simulink library "GAS_MASTER"  (Simulink 8.6)
settings: Solver=ode45  StartTime=0.0  StopTime=10.0  RelTol=1e-3
libraries: cdsEpicsOut x24, cdsFilt x14, cdsFiltCtrl x10, cdsTP x8, VIS_LIB x8, cdsEpicsBinIn x7, cdsEpicsIn x6, cdsFunctionCall x4
(part 1 of 3)
settings Model: Creator=controls  LastModifiedBy=controls

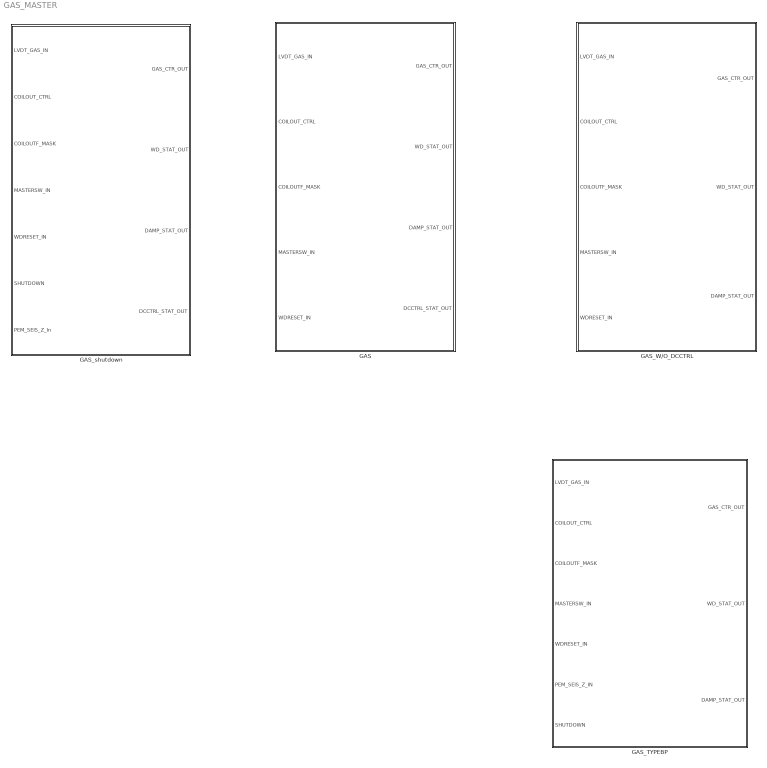
== system GAS_MASTER ==
  GAS : Subsystem
  GAS_TYPEBP : Subsystem
  GAS_W/O_DCCTRL : Subsystem
  GAS_shutdown : Subsystem

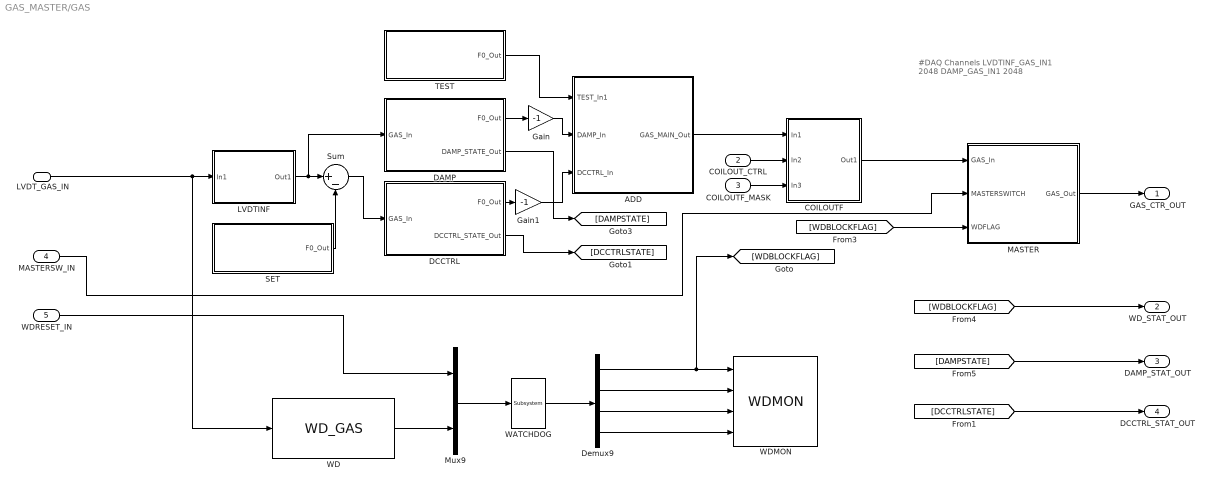
== system GAS_MASTER/GAS ==
  note: #DAQ Channels
      | LVDTINF_GAS_IN1 2048
      | DAMP_GAS_IN1 2048
  LVDT_GAS_IN : Inport
  COILOUT_CTRL : Inport  Port=2
  COILOUTF_MASK : Inport  Port=3
  MASTERSW_IN : Inport  Port=4
  WDRESET_IN : Inport  Port=5
  ADD : Subsystem
  COILOUTF : Subsystem
  DAMP : Subsystem
  DCCTRL : Subsystem
  Demux9 : Demux
  Gain : Gain  Gain=-1
  Gain1 : Gain  Gain=-1
  LVDTINF : Subsystem
  MASTER : Subsystem
  Mux9 : Mux  Inputs=2
  SET : Subsystem
  Sum : Sum  Inputs=|+-
  TEST : Subsystem
  WATCHDOG : cdsFunctionCall/Subsystem  Tag=cdsFunctionCall  Description=inline OSEMWATCHDOG /opt/rtcds/userapps/release/vis/common/src/WATCHDOG.c
      settings: AttributesFormatString=%<Tag>\n%<Description>
  WD : VIS_LIB/WD_GAS
  WDMON : VIS_LIB/WDMON
  GAS_CTR_OUT : Outport
  WD_STAT_OUT : Outport  Port=2
  DAMP_STAT_OUT : Outport  Port=3
  DCCTRL_STAT_OUT : Outport  Port=4
  wires:
  Demux9/2 -> WDMON/2
  Demux9/3 -> WDMON/3
  WD/1 -> Mux9/2
  COILOUTF/1(Out1) -> MASTER/1(GAS_In)
  LVDTINF/1(Out1) -> Sum/1, DAMP/1(GAS_In)
  WATCHDOG/1 -> Demux9/1
  Demux9/4 -> WDMON/4
  Mux9/1 -> WATCHDOG/1
  DAMP/2(DAMP_STATE_Out) -> [DAMPSTATE]
  DAMP/1(F0_Out) -> Gain/1
  MASTERSW_IN/1 -> MASTER/2(MASTERSWITCH)
  [WDBLOCKFLAG] -> WD_STAT_OUT/1
  [DAMPSTATE] -> DAMP_STAT_OUT/1
  [WDBLOCKFLAG] -> MASTER/3(WDFLAG)
  MASTER/1(GAS_Out) -> GAS_CTR_OUT/1
  ADD/1(GAS_MAIN_Out) -> COILOUTF/1(In1)
  Demux9/1 -> [WDBLOCKFLAG], WDMON/1
  LVDT_GAS_IN/1 -> LVDTINF/1(In1), WD/1
  COILOUT_CTRL/1 -> COILOUTF/2(In2)
  COILOUTF_MASK/1 -> COILOUTF/3(In3)
  WDRESET_IN/1 -> Mux9/1
  DCCTRL/1(F0_Out) -> Gain1/1
  DCCTRL/2(DCCTRL_STATE_Out) -> [DCCTRLSTATE]
  [DCCTRLSTATE] -> DCCTRL_STAT_OUT/1
  Sum/1 -> DCCTRL/1(GAS_In)
  TEST/1(F0_Out) -> ADD/1(TEST_In1)
  Gain/1 -> ADD/2(DAMP_In)
  Gain1/1 -> ADD/3(DCCTRL_In)
  SET/1(F0_Out) -> Sum/2

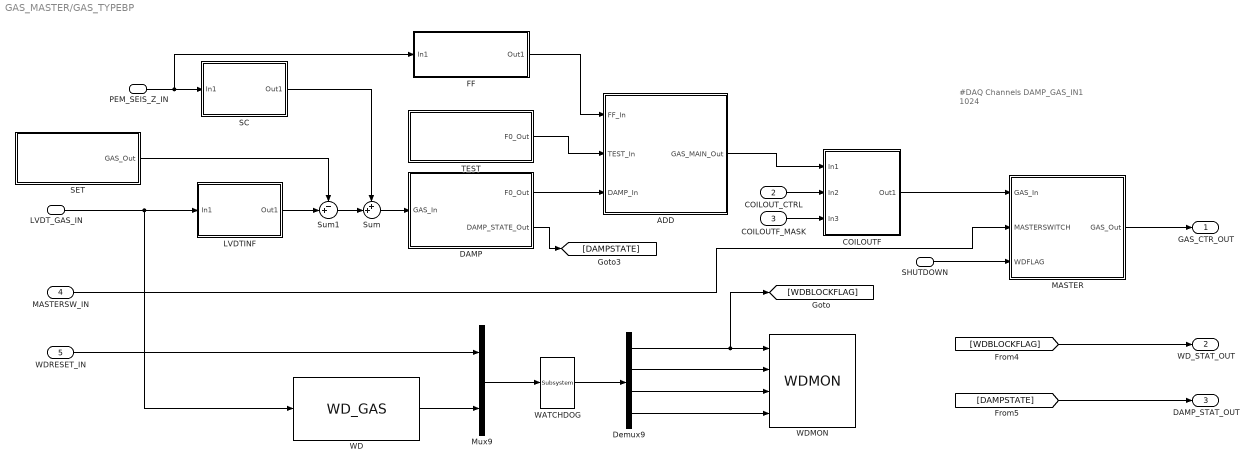
== system GAS_MASTER/GAS_TYPEBP ==
  note: #DAQ Channels
      | DAMP_GAS_IN1 1024
  LVDT_GAS_IN : Inport
  COILOUT_CTRL : Inport  Port=2
  COILOUTF_MASK : Inport  Port=3
  MASTERSW_IN : Inport  Port=4
  WDRESET_IN : Inport  Port=5
  PEM_SEIS_Z_IN : Inport  Port=6
  SHUTDOWN : Inport  Port=7
  ADD : Subsystem
  COILOUTF : Subsystem
  DAMP : Subsystem
  Demux9 : Demux
  FF : Subsystem
  LVDTINF : Subsystem
  MASTER : Subsystem
  Mux9 : Mux  Inputs=2
  SC : Subsystem
  SET : Subsystem
  Sum : Sum  Inputs=++|
  Sum1 : Sum  Inputs=-+|
  TEST : Subsystem
  WATCHDOG : cdsFunctionCall/Subsystem  Tag=cdsFunctionCall  Description=inline OSEMWATCHDOG /opt/rtcds/userapps/release/vis/common/src/WATCHDOG.c
      settings: AttributesFormatString=%<Tag>\n%<Description>
  WD : VIS_LIB/WD_GAS
  WDMON : VIS_LIB/WDMON
  GAS_CTR_OUT : Outport
  WD_STAT_OUT : Outport  Port=2
  DAMP_STAT_OUT : Outport  Port=3
  wires:
  Demux9/2 -> WDMON/2
  Demux9/3 -> WDMON/3
  WD/1 -> Mux9/2
  COILOUTF/1(Out1) -> MASTER/1(GAS_In)
  WATCHDOG/1 -> Demux9/1
  Demux9/4 -> WDMON/4
  Mux9/1 -> WATCHDOG/1
  DAMP/2(DAMP_STATE_Out) -> [DAMPSTATE]
  DAMP/1(F0_Out) -> ADD/3(DAMP_In)
  MASTERSW_IN/1 -> MASTER/2(MASTERSWITCH)
  [WDBLOCKFLAG] -> WD_STAT_OUT/1
  [DAMPSTATE] -> DAMP_STAT_OUT/1
  TEST/1(F0_Out) -> ADD/2(TEST_In)
  SHUTDOWN/1 -> MASTER/3(WDFLAG)
  MASTER/1(GAS_Out) -> GAS_CTR_OUT/1
  ADD/1(GAS_MAIN_Out) -> COILOUTF/1(In1)
  Demux9/1 -> [WDBLOCKFLAG], WDMON/1
  LVDT_GAS_IN/1 -> LVDTINF/1(In1), WD/1
  COILOUT_CTRL/1 -> COILOUTF/2(In2)
  COILOUTF_MASK/1 -> COILOUTF/3(In3)
  WDRESET_IN/1 -> Mux9/1
  PEM_SEIS_Z_IN/1 -> FF/1(In1), SC/1(In1)
  SC/1(Out1) -> Sum/1
  Sum/1 -> DAMP/1(GAS_In)
  FF/1(Out1) -> ADD/1(FF_In)
  LVDTINF/1(Out1) -> Sum1/2
  Sum1/1 -> Sum/2
  SET/1(GAS_Out) -> Sum1/1

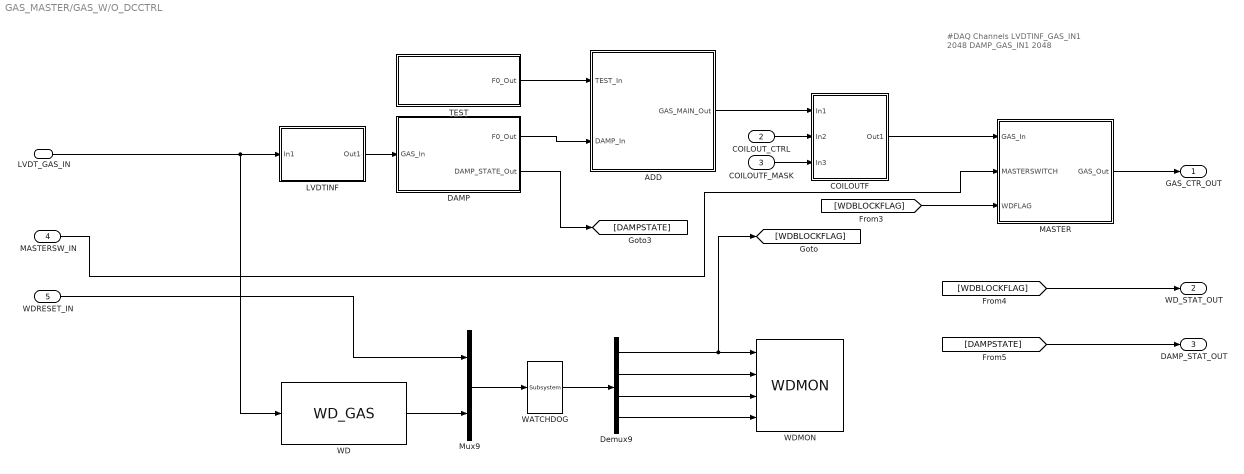
== system GAS_MASTER/GAS_W/O_DCCTRL ==
  note: #DAQ Channels
      | LVDTINF_GAS_IN1 2048
      | DAMP_GAS_IN1 2048
  LVDT_GAS_IN : Inport
  COILOUT_CTRL : Inport  Port=2
  COILOUTF_MASK : Inport  Port=3
  MASTERSW_IN : Inport  Port=4
  WDRESET_IN : Inport  Port=5
  ADD : Subsystem
  COILOUTF : Subsystem
  DAMP : Subsystem
  Demux9 : Demux
  LVDTINF : Subsystem
  MASTER : Subsystem
  Mux9 : Mux  Inputs=2
  TEST : Subsystem
  WATCHDOG : cdsFunctionCall/Subsystem  Tag=cdsFunctionCall  Description=inline OSEMWATCHDOG /opt/rtcds/userapps/release/vis/common/src/WATCHDOG.c
      settings: AttributesFormatString=%<Tag>\n%<Description>
  WD : VIS_LIB/WD_GAS
  WDMON : VIS_LIB/WDMON
  GAS_CTR_OUT : Outport
  WD_STAT_OUT : Outport  Port=2
  DAMP_STAT_OUT : Outport  Port=3
  wires:
  Demux9/2 -> WDMON/2
  Demux9/3 -> WDMON/3
  WD/1 -> Mux9/2
  COILOUTF/1(Out1) -> MASTER/1(GAS_In)
  LVDTINF/1(Out1) -> DAMP/1(GAS_In)
  WATCHDOG/1 -> Demux9/1
  Demux9/4 -> WDMON/4
  Mux9/1 -> WATCHDOG/1
  DAMP/2(DAMP_STATE_Out) -> [DAMPSTATE]
  DAMP/1(F0_Out) -> ADD/2(DAMP_In)
  MASTERSW_IN/1 -> MASTER/2(MASTERSWITCH)
  [WDBLOCKFLAG] -> WD_STAT_OUT/1
  [DAMPSTATE] -> DAMP_STAT_OUT/1
  TEST/1(F0_Out) -> ADD/1(TEST_In)
  [WDBLOCKFLAG] -> MASTER/3(WDFLAG)
  MASTER/1(GAS_Out) -> GAS_CTR_OUT/1
  ADD/1(GAS_MAIN_Out) -> COILOUTF/1(In1)
  Demux9/1 -> [WDBLOCKFLAG], WDMON/1
  LVDT_GAS_IN/1 -> WD/1, LVDTINF/1(In1)
  COILOUT_CTRL/1 -> COILOUTF/2(In2)
  COILOUTF_MASK/1 -> COILOUTF/3(In3)
  WDRESET_IN/1 -> Mux9/1

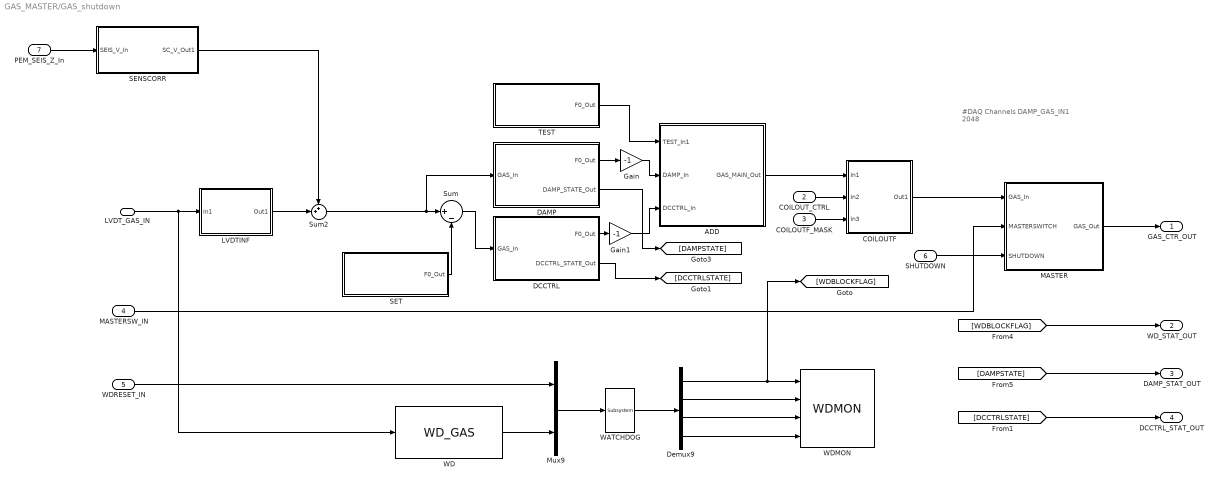
== system GAS_MASTER/GAS_shutdown ==
  note: #DAQ Channels
      | DAMP_GAS_IN1 2048
  LVDT_GAS_IN : Inport
  COILOUT_CTRL : Inport  Port=2
  COILOUTF_MASK : Inport  Port=3
  MASTERSW_IN : Inport  Port=4
  WDRESET_IN : Inport  Port=5
  SHUTDOWN : Inport  Port=6
  PEM_SEIS_Z_In : Inport  Port=7
  ADD : Subsystem
  COILOUTF : Subsystem
  DAMP : Subsystem
  DCCTRL : Subsystem
  Demux9 : Demux
  Gain : Gain  Gain=-1
  Gain1 : Gain  Gain=-1
  LVDTINF : Subsystem
  MASTER : Subsystem
  Mux9 : Mux  Inputs=2
  SENSCORR : Subsystem
  SET : Subsystem
  Sum : Sum  Inputs=|+-
  Sum2 : Sum  Inputs=++|
  TEST : Subsystem
  WATCHDOG : cdsFunctionCall/Subsystem  Tag=cdsFunctionCall  Description=inline OSEMWATCHDOG /opt/rtcds/userapps/release/vis/common/src/WATCHDOG.c
      settings: AttributesFormatString=%<Tag>\n%<Description>
  WD : VIS_LIB/WD_GAS
  WDMON : VIS_LIB/WDMON
  GAS_CTR_OUT : Outport
  WD_STAT_OUT : Outport  Port=2
  DAMP_STAT_OUT : Outport  Port=3
  DCCTRL_STAT_OUT : Outport  Port=4
  wires:
  LVDTINF/1(Out1) -> Sum2/2
  SENSCORR/1(SC_V_Out1) -> Sum2/1
  PEM_SEIS_Z_In/1 -> SENSCORR/1(SEIS_V_In)
  Demux9/2 -> WDMON/2
  Demux9/3 -> WDMON/3
  WD/1 -> Mux9/2
  COILOUTF/1(Out1) -> MASTER/1(GAS_In)
  Sum2/1 -> Sum/1, DAMP/1(GAS_In)
  WATCHDOG/1 -> Demux9/1
  Demux9/4 -> WDMON/4
  Mux9/1 -> WATCHDOG/1
  DAMP/2(DAMP_STATE_Out) -> [DAMPSTATE]
  DAMP/1(F0_Out) -> Gain/1
  MASTERSW_IN/1 -> MASTER/2(MASTERSWITCH)
  [WDBLOCKFLAG] -> WD_STAT_OUT/1
  [DAMPSTATE] -> DAMP_STAT_OUT/1
  SHUTDOWN/1 -> MASTER/3(SHUTDOWN)
  MASTER/1(GAS_Out) -> GAS_CTR_OUT/1
  ADD/1(GAS_MAIN_Out) -> COILOUTF/1(In1)
  Demux9/1 -> [WDBLOCKFLAG], WDMON/1
  LVDT_GAS_IN/1 -> WD/1, LVDTINF/1(In1)
  COILOUT_CTRL/1 -> COILOUTF/2(In2)
  COILOUTF_MASK/1 -> COILOUTF/3(In3)
  WDRESET_IN/1 -> Mux9/1
  DCCTRL/1(F0_Out) -> Gain1/1
  DCCTRL/2(DCCTRL_STATE_Out) -> [DCCTRLSTATE]
  [DCCTRLSTATE] -> DCCTRL_STAT_OUT/1
  Sum/1 -> DCCTRL/1(GAS_In)
  TEST/1(F0_Out) -> ADD/1(TEST_In1)
  Gain/1 -> ADD/2(DAMP_In)
  Gain1/1 -> ADD/3(DCCTRL_In)
  SET/1(F0_Out) -> Sum/2

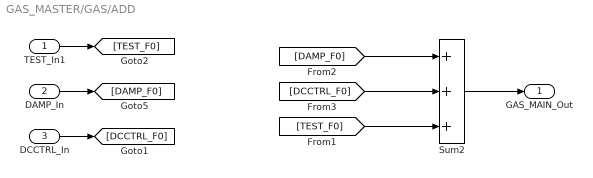
== system GAS_MASTER/GAS/ADD ==
  TEST_In1 : Inport
  DAMP_In : Inport  Port=2
  DCCTRL_In : Inport  Port=3
  Sum2 : Sum  Inputs=+++
  GAS_MAIN_Out : Outport
  wires:
  [DAMP_F0] -> Sum2/1
  Sum2/1 -> GAS_MAIN_Out/1
  DAMP_In/1 -> [DAMP_F0]
  [DCCTRL_F0] -> Sum2/2
  DCCTRL_In/1 -> [DCCTRL_F0]
  TEST_In1/1 -> [TEST_F0]
  [TEST_F0] -> Sum2/3

== system GAS_MASTER/GAS/COILOUTF ==
  In1 : Inport
  In2 : Inport  Port=2
  In3 : Inport  Port=3
  GAS : cdsFiltCtrl/IIR FM with control  Tag=cdsFiltCtrl  Description=|
      | cdsFiltCntrl is the standard IIR filter module (exactly the same as cdsFilt) but with added control data output 'Ctrl'. Filter module digital signal output appears on the first output, which is called 'Val'. 'Ctrl' output has a bit pattern encoding the state of filter's on/off switches (FM1 through FM10). The bit values are:
      |                                                                                                                                                                                                                                                                                                                                       
      | module 	hex	dec                                                                                                                                                                                                                                                                                                                       
      | -----------------------                                                                                                                                                                                                                                                                                                               
      | FM1	0x20                    32                                                                                                                                                                                                                                                                                                        
      | FM2	0x80                     128                                                                                                                                                                                                                                                                                                      
      | FM3	0x200                   512                                                                                                                                                                                                                                                                                                       
      | FM4	0x800                   2048                                                                                                                                                                                                                                                                                                      
      | FM5	0x2000                 8192                                                                                                                                                                                                                                                                                                       
      | FM6	0x8000                 32768                                                                                                                                                                                                                                                                                                      
      | FM7	0x20000                131072                                                                                                                                                                                                                                                                                                     
      | FM8	0x80000                 524288                                                                                                                                                                                                                                                                                                    
      | FM9	0x200000               2097152                                                                                                                                                                                                                                                                                                    
      | FM10	0x800000               8388608                                                                                                                                                                                                                                                                                                   
      |                                                                                                                                                                                                                                                                                                                                       
      | This bit data can be used to drive some other switches or it can be output using a binary I/O module.
      settings: AttributesFormatString=%<Tag>
  Out1 : Outport
  wires:
  GAS/1 -> Out1/1
  In2/1 -> GAS/2
  In3/1 -> GAS/3
  In1/1 -> GAS/1

== system GAS_MASTER/GAS/DAMP ==
  note: 1 (one) if GOOD
      | 0 (zero) if BAD
  note: Each DAMP filter output bitword is
      | compared against a known good state.
      | If equal to good state, then a 1 is output
      | and multiplied into the product. So, if any DOF
      | is not in its good state, the whole product is 0.
  GAS_In : Inport
  GAS : cdsFiltCtrl/IIR FM with control  Tag=cdsFiltCtrl  Description=|
      | cdsFiltCntrl is the standard IIR filter module (exactly the same as cdsFilt) but with added control data output 'Ctrl'. Filter module digital signal output appears on the first output, which is called 'Val'. 'Ctrl' output has a bit pattern encoding the state of filter's on/off switches (FM1 through FM10). The bit values are:
      |                                                                                                                                                                                                                                                                                                                                       
      | module 	hex	dec                                                                                                                                                                                                                                                                                                                       
      | -----------------------                                                                                                                                                                                                                                                                                                               
      | FM1	0x20                    32                                                                                                                                                                                                                                                                                                        
      | FM2	0x80                     128                                                                                                                                                                                                                                                                                                      
      | FM3	0x200                   512                                                                                                                                                                                                                                                                                                       
      | FM4	0x800                   2048                                                                                                                                                                                                                                                                                                      
      | FM5	0x2000                 8192                                                                                                                                                                                                                                                                                                       
      | FM6	0x8000                 32768                                                                                                                                                                                                                                                                                                      
      | FM7	0x20000                131072                                                                                                                                                                                                                                                                                                     
      | FM8	0x80000                 524288                                                                                                                                                                                                                                                                                                    
      | FM9	0x200000               2097152                                                                                                                                                                                                                                                                                                    
      | FM10	0x800000               8388608                                                                                                                                                                                                                                                                                                   
      |                                                                                                                                                                                                                                                                                                                                       
      | This bit data can be used to drive some other switches or it can be output using a binary I/O module.
      settings: AttributesFormatString=%<Tag>
  GAS_STATE_GOOD : cdsEpicsIn/Subsystem  Tag=cdsEpicsIn  Description=|
      | Purpose:                                                                              
      | Create an EPICS input channel connection to the FE realtime controls.                 
      |                                                                                       
      | Operation:                                                                            
      | Outputs value from an EPICS ai record. Value is floating point with a precision of 3..
      |                                                                                       
      | Usage:                                                                                
      | Name the part with the desired EPICS channel name.
      settings: AttributesFormatString=%<Tag>
  GAS_STATE_NOW : cdsEpicsOut/Subsystem  Tag=cdsEpicsOutput  Description=|
      | Purpose:                                          
      | Output a FE signal to an EPICS channel.           
      |                                                   
      | Operation:                                        
      | Takes input value and passes it to EPICS record.  
      |                                                   
      | Usage:                                            
      | Name the part with the desired EPICS rrecord name.
      settings: AttributesFormatString=%<Tag>
  Ground6 : Ground
  Ground8 : Ground
  Operator : RelationalOperator  Operator===  OutDataTypeStr=boolean
  STATE_OK : cdsEpicsOut/Subsystem  Tag=cdsEpicsOutput  Description=|
      | Purpose:                                          
      | Output a FE signal to an EPICS channel.           
      |                                                   
      | Operation:                                        
      | Takes input value and passes it to EPICS record.  
      |                                                   
      | Usage:                                            
      | Name the part with the desired EPICS rrecord name.
      settings: AttributesFormatString=%<Tag>
  F0_Out : Outport
  DAMP_STATE_Out : Outport  Port=2
  wires:
  Operator/1 -> STATE_OK/1
  Ground8/1 -> GAS/3
  STATE_OK/1 -> DAMP_STATE_Out/1
  GAS_STATE_NOW/1 -> Operator/2
  GAS/2 -> GAS_STATE_NOW/1
  GAS_STATE_GOOD/1 -> Operator/1
  GAS/1 -> F0_Out/1
  GAS_In/1 -> GAS/1
  Ground6/1 -> GAS/2

== system GAS_MASTER/GAS/DCCTRL ==
  note: 1 (one) if GOOD
      | 0 (zero) if BAD
  note: Each DAMP filter output bitword is
      | compared against a known good state.
      | If equal to good state, then a 1 is output
      | and multiplied into the product. So, if any DOF
      | is not in its good state, the whole product is 0.
  GAS_In : Inport
  GAS : cdsFiltCtrl/IIR FM with control  Tag=cdsFiltCtrl  Description=|
      | cdsFiltCntrl is the standard IIR filter module (exactly the same as cdsFilt) but with added control data output 'Ctrl'. Filter module digital signal output appears on the first output, which is called 'Val'. 'Ctrl' output has a bit pattern encoding the state of filter's on/off switches (FM1 through FM10). The bit values are:
      |                                                                                                                                                                                                                                                                                                                                       
      | module 	hex	dec                                                                                                                                                                                                                                                                                                                       
      | -----------------------                                                                                                                                                                                                                                                                                                               
      | FM1	0x20                    32                                                                                                                                                                                                                                                                                                        
      | FM2	0x80                     128                                                                                                                                                                                                                                                                                                      
      | FM3	0x200                   512                                                                                                                                                                                                                                                                                                       
      | FM4	0x800                   2048                                                                                                                                                                                                                                                                                                      
      | FM5	0x2000                 8192                                                                                                                                                                                                                                                                                                       
      | FM6	0x8000                 32768                                                                                                                                                                                                                                                                                                      
      | FM7	0x20000                131072                                                                                                                                                                                                                                                                                                     
      | FM8	0x80000                 524288                                                                                                                                                                                                                                                                                                    
      | FM9	0x200000               2097152                                                                                                                                                                                                                                                                                                    
      | FM10	0x800000               8388608                                                                                                                                                                                                                                                                                                   
      |                                                                                                                                                                                                                                                                                                                                       
      | This bit data can be used to drive some other switches or it can be output using a binary I/O module.
      settings: AttributesFormatString=%<Tag>
  GAS_STATE_GOOD : cdsEpicsIn/Subsystem  Tag=cdsEpicsIn  Description=|
      | Purpose:                                                                              
      | Create an EPICS input channel connection to the FE realtime controls.                 
      |                                                                                       
      | Operation:                                                                            
      | Outputs value from an EPICS ai record. Value is floating point with a precision of 3..
      |                                                                                       
      | Usage:                                                                                
      | Name the part with the desired EPICS channel name.
      settings: AttributesFormatString=%<Tag>
  GAS_STATE_NOW : cdsEpicsOut/Subsystem  Tag=cdsEpicsOutput  Description=|
      | Purpose:                                          
      | Output a FE signal to an EPICS channel.           
      |                                                   
      | Operation:                                        
      | Takes input value and passes it to EPICS record.  
      |                                                   
      | Usage:                                            
      | Name the part with the desired EPICS rrecord name.
      settings: AttributesFormatString=%<Tag>
  Ground6 : Ground
  Ground8 : Ground
  Operator : RelationalOperator  Operator===  OutDataTypeStr=boolean
  STATE_OK : cdsEpicsOut/Subsystem  Tag=cdsEpicsOutput  Description=|
      | Purpose:                                          
      | Output a FE signal to an EPICS channel.           
      |                                                   
      | Operation:                                        
      | Takes input value and passes it to EPICS record.  
      |                                                   
      | Usage:                                            
      | Name the part with the desired EPICS rrecord name.
      settings: AttributesFormatString=%<Tag>
  F0_Out : Outport
  DCCTRL_STATE_Out : Outport  Port=2
  wires:
  Operator/1 -> STATE_OK/1
  Ground8/1 -> GAS/3
  STATE_OK/1 -> DCCTRL_STATE_Out/1
  GAS_STATE_NOW/1 -> Operator/2
  GAS/2 -> GAS_STATE_NOW/1
  GAS_STATE_GOOD/1 -> Operator/1
  GAS/1 -> F0_Out/1
  GAS_In/1 -> GAS/1
  Ground6/1 -> GAS/2

== system GAS_MASTER/GAS/LVDTINF ==
  In1 : Inport
  GAS : cdsFilt/Subsystem  Tag=cdsFilt  Description=|
      | Purpose:                                                                                                                                                                                                                                  
      | Standard CDS IIR filter module.                                                                                                                                                                                                           
      |                                                                                                                                                                                                                                           
      | Operation:                                                                                                                                                                                                                                
      | Consists of 10 second order section IIR filters, plus a ramped gain stage. In FE code, also provides pre-defined test points and excitation channel inputs. The filter coefficients are defined in the LIGO system using the 'foton' tool.
      |                                                                                                                                                                                                                                           
      | Usage:                                                                                                                                                                                                                                    
      | Name the part with the desired filter module name.
      settings: AttributesFormatString=%<Tag>
  Out1 : Outport
  wires:
  GAS/1 -> Out1/1
  In1/1 -> GAS/1

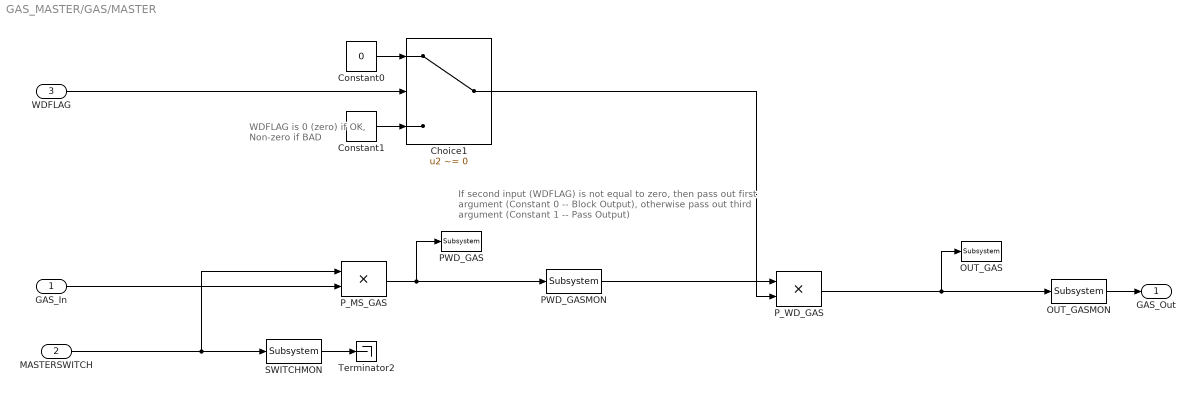
== system GAS_MASTER/GAS/MASTER ==
  note: If second input (WDFLAG) is not equal to zero,
      | then pass out first argument (Constant 0 -- Block Output),
      | otherwise pass out third argument (Constant 1 -- Pass Output)
  note: WDFLAG is 0 (zero) if OK,
      | Non-zero if BAD
  GAS_In : Inport
  MASTERSWITCH : Inport  Port=2
  WDFLAG : Inport  Port=3
  Choice1 : Switch  Criteria=u2 ~= 0  Threshold=0.5
  Constant0 : Constant  Value=0
  Constant1 : Constant
  OUT_GAS : cdsTP/Subsystem  Tag=Test Point
      settings: AttributesFormatString=%<Tag>
  OUT_GASMON : cdsEpicsOut/Subsystem  Tag=cdsEpicsOutput  Description=|
      | Purpose:                                          
      | Output a FE signal to an EPICS channel.           
      |                                                   
      | Operation:                                        
      | Takes input value and passes it to EPICS record.  
      |                                                   
      | Usage:                                            
      | Name the part with the desired EPICS rrecord name.
      settings: AttributesFormatString=%<Tag>
  PWD_GAS : cdsTP/Subsystem  Tag=Test Point
      settings: AttributesFormatString=%<Tag>
  PWD_GASMON : cdsEpicsOut/Subsystem  Tag=cdsEpicsOutput  Description=|
      | Purpose:                                          
      | Output a FE signal to an EPICS channel.           
      |                                                   
      | Operation:                                        
      | Takes input value and passes it to EPICS record.  
      |                                                   
      | Usage:                                            
      | Name the part with the desired EPICS rrecord name.
      settings: AttributesFormatString=%<Tag>
  P_MS_GAS : Product  RndMeth=Zero
  P_WD_GAS : Product  RndMeth=Zero
  SWITCHMON : cdsEpicsOut/Subsystem  Tag=cdsEpicsOutput  Description=|
      | Purpose:                                          
      | Output a FE signal to an EPICS channel.           
      |                                                   
      | Operation:                                        
      | Takes input value and passes it to EPICS record.  
      |                                                   
      | Usage:                                            
      | Name the part with the desired EPICS rrecord name.
      settings: AttributesFormatString=%<Tag>
  Terminator2 : Terminator
  GAS_Out : Outport
  wires:
  SWITCHMON/1 -> Terminator2/1
  GAS_In/1 -> P_MS_GAS/2
  MASTERSWITCH/1 -> SWITCHMON/1, P_MS_GAS/1
  OUT_GASMON/1 -> GAS_Out/1
  P_MS_GAS/1 -> PWD_GAS/1, PWD_GASMON/1
  P_WD_GAS/1 -> OUT_GASMON/1, OUT_GAS/1
  Constant1/1 -> Choice1/3
  Constant0/1 -> Choice1/1
  WDFLAG/1 -> Choice1/2
  PWD_GASMON/1 -> P_WD_GAS/1
  Choice1/1 -> P_WD_GAS/2

== system GAS_MASTER/GAS/SET ==
  GAS : cdsFilt/Subsystem  Tag=cdsFilt  Description=|
      | Purpose:                                                                                                                                                                                                                                  
      | Standard CDS IIR filter module.                                                                                                                                                                                                           
      |                                                                                                                                                                                                                                           
      | Operation:                                                                                                                                                                                                                                
      | Consists of 10 second order section IIR filters, plus a ramped gain stage. In FE code, also provides pre-defined test points and excitation channel inputs. The filter coefficients are defined in the LIGO system using the 'foton' tool.
      |                                                                                                                                                                                                                                           
      | Usage:                                                                                                                                                                                                                                    
      | Name the part with the desired filter module name.
      settings: AttributesFormatString=%<Tag>
  Ground1 : Ground
  Ground7 : Ground
  STATUS : cdsEpicsBinIn/Subsystem  Tag=cdsEpicsBinIn  Description=|
      | Purpose:                                                                            
      | Create an EPICS binary (0 or 1) input channel to the FE realtime controls.          
      |                                                                                     
      | Operation:                                                                          
      | Outputs value from an EPICS ai record. Value is binary input (bi Epics record type).
      |                                                                                     
      | Usage:                                                                              
      | Name the part with the desired EPICS channel name.
      settings: AttributesFormatString=%<Tag>
  F0_Out : Outport
  wires:
  GAS/1 -> F0_Out/1
  Ground1/1 -> GAS/1
  Ground7/1 -> STATUS/1

== system GAS_MASTER/GAS/TEST ==
  GAS : cdsFilt/Subsystem  Tag=cdsFilt  Description=|
      | Purpose:                                                                                                                                                                                                                                  
      | Standard CDS IIR filter module.                                                                                                                                                                                                           
      |                                                                                                                                                                                                                                           
      | Operation:                                                                                                                                                                                                                                
      | Consists of 10 second order section IIR filters, plus a ramped gain stage. In FE code, also provides pre-defined test points and excitation channel inputs. The filter coefficients are defined in the LIGO system using the 'foton' tool.
      |                                                                                                                                                                                                                                           
      | Usage:                                                                                                                                                                                                                                    
      | Name the part with the desired filter module name.
      settings: AttributesFormatString=%<Tag>
  Ground1 : Ground
  Ground7 : Ground
  STATUS : cdsEpicsBinIn/Subsystem  Tag=cdsEpicsBinIn  Description=|
      | Purpose:                                                                            
      | Create an EPICS binary (0 or 1) input channel to the FE realtime controls.          
      |                                                                                     
      | Operation:                                                                          
      | Outputs value from an EPICS ai record. Value is binary input (bi Epics record type).
      |                                                                                     
      | Usage:                                                                              
      | Name the part with the desired EPICS channel name.
      settings: AttributesFormatString=%<Tag>
  F0_Out : Outport
  wires:
  GAS/1 -> F0_Out/1
  Ground1/1 -> GAS/1
  Ground7/1 -> STATUS/1

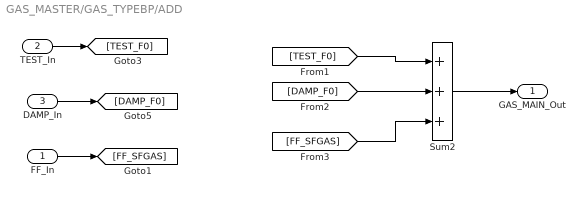
== system GAS_MASTER/GAS_TYPEBP/ADD ==
  FF_In : Inport
  TEST_In : Inport  Port=2
  DAMP_In : Inport  Port=3
  Sum2 : Sum  Inputs=+++
  GAS_MAIN_Out : Outport
  wires:
  [DAMP_F0] -> Sum2/2
  [TEST_F0] -> Sum2/1
  Sum2/1 -> GAS_MAIN_Out/1
  TEST_In/1 -> [TEST_F0]
  DAMP_In/1 -> [DAMP_F0]
  FF_In/1 -> [FF_SFGAS]
  [FF_SFGAS] -> Sum2/3

== system GAS_MASTER/GAS_TYPEBP/COILOUTF ==
  In1 : Inport
  In2 : Inport  Port=2
  In3 : Inport  Port=3
  GAS : cdsFiltCtrl/IIR FM with control  Tag=cdsFiltCtrl  Description=|
      | cdsFiltCntrl is the standard IIR filter module (exactly the same as cdsFilt) but with added control data output 'Ctrl'. Filter module digital signal output appears on the first output, which is called 'Val'. 'Ctrl' output has a bit pattern encoding the state of filter's on/off switches (FM1 through FM10). The bit values are:
      |                                                                                                                                                                                                                                                                                                                                       
      | module 	hex	dec                                                                                                                                                                                                                                                                                                                       
      | -----------------------                                                                                                                                                                                                                                                                                                               
      | FM1	0x20                    32                                                                                                                                                                                                                                                                                                        
      | FM2	0x80                     128                                                                                                                                                                                                                                                                                                      
      | FM3	0x200                   512                                                                                                                                                                                                                                                                                                       
      | FM4	0x800                   2048                                                                                                                                                                                                                                                                                                      
      | FM5	0x2000                 8192                                                                                                                                                                                                                                                                                                       
      | FM6	0x8000                 32768                                                                                                                                                                                                                                                                                                      
      | FM7	0x20000                131072                                                                                                                                                                                                                                                                                                     
      | FM8	0x80000                 524288                                                                                                                                                                                                                                                                                                    
      | FM9	0x200000               2097152                                                                                                                                                                                                                                                                                                    
      | FM10	0x800000               8388608                                                                                                                                                                                                                                                                                                   
      |                                                                                                                                                                                                                                                                                                                                       
      | This bit data can be used to drive some other switches or it can be output using a binary I/O module.
      settings: AttributesFormatString=%<Tag>
  Out1 : Outport
  wires:
  GAS/1 -> Out1/1
  In2/1 -> GAS/2
  In3/1 -> GAS/3
  In1/1 -> GAS/1
